simulink model "exercise1_Dengliang"  (R2024b)
settings: Solver=VariableStepAuto  StartTime=0.0  StopTime=20000  RelTol=1e-3
libraries: simulink x4
settings Model: Creator=10027  LastModifiedBy=10027

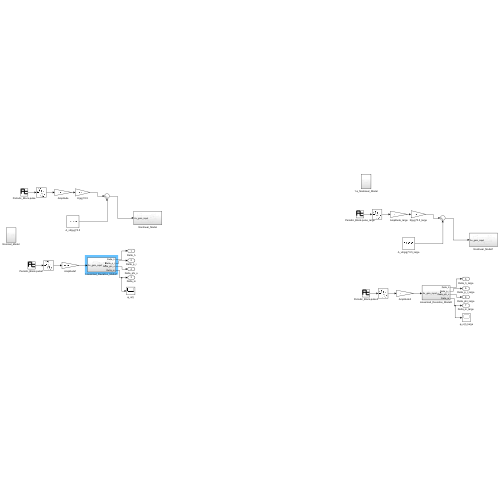
[thumbnail: Simulink's stored preview of the top-level diagram]
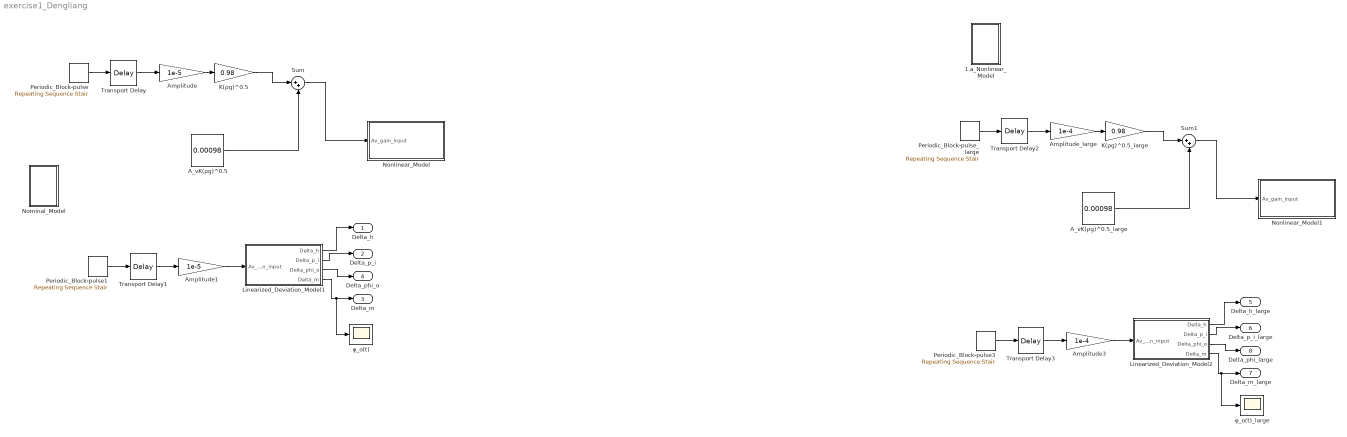
== system exercise1_Dengliang ==
  1.a_Nonlinear_Model : Subsystem
  A_vK(ρg)^0.5 : Constant  Value=0.00098
  A_vK(ρg)^0.5_large : Constant  Value=0.00098
  Amplitude : Gain  Gain=1e-5
  Amplitude1 : Gain  Gain=1e-5
  Amplitude3 : Gain  Gain=1e-4
  Amplitude_large : Gain  Gain=1e-4
  K(ρg)^0.5 : Gain  Gain=0.98
  K(ρg)^0.5_large : Gain  Gain=0.98
  Linearized_Deviation_Model1 : Subsystem
  Linearized_Deviation_Model2 : Subsystem
  Nominal_Model : Subsystem
  Nonlinear_Model : Subsystem
  Nonlinear_Model1 : Subsystem
  Periodic_Block-pulse : simulink/Sources/Repeating Sequence Stair  OutValues=[1 -1]  tsamp=3000  OutMin=[]  OutMax=[]  OutDataTypeStr=double  OutputDataTypeScalingMode=double  OutDataType=fixdt(0,8)  ConRadixGroup=Best Precision: Vector-wise  OutScaling=2^-12
  Periodic_Block-pulse1 : simulink/Sources/Repeating Sequence Stair  OutValues=[1 -1]  tsamp=3000  OutMin=[]  OutMax=[]  OutDataTypeStr=double  OutputDataTypeScalingMode=double  OutDataType=fixdt(0,8)  ConRadixGroup=Best Precision: Vector-wise  OutScaling=2^-12
  Periodic_Block-pulse3 : simulink/Sources/Repeating Sequence Stair  OutValues=[1 -1]  tsamp=3000  OutMin=[]  OutMax=[]  OutDataTypeStr=double  OutputDataTypeScalingMode=double  OutDataType=fixdt(0,8)  ConRadixGroup=Best Precision: Vector-wise  OutScaling=2^-12
  Periodic_Block-pulse_large : simulink/Sources/Repeating Sequence Stair  OutValues=[1 -1]  tsamp=3000  OutMin=[]  OutMax=[]  OutDataTypeStr=double  OutputDataTypeScalingMode=double  OutDataType=fixdt(0,8)  ConRadixGroup=Best Precision: Vector-wise  OutScaling=2^-12
  Sum : Sum  Inputs=|++
  Sum1 : Sum  Inputs=|++
  Transport Delay{,1..3} (4 alike) : TransportDelay  DelayTime=1000
  φ_o(t) : Scope
  φ_o(t)_large : Scope
  Delta_h : Outport
  Delta_p_i : Outport  Port=2
  Delta_m : Outport  Port=3
  Delta_phi_o : Outport  Port=4
  Delta_h_large : Outport  Port=5
  Delta_p_i_large : Outport  Port=6
  Delta_m_large : Outport  Port=7
  Delta_phi_large : Outport  Port=8
  wires:
  Periodic_Block-pulse/1 -> Transport Delay/1
  Amplitude/1 -> K(ρg)^0.5/1
  Transport Delay/1 -> Amplitude/1
  K(ρg)^0.5/1 -> Sum/1
  Sum/1 -> Nonlinear_Model/1(Av_gain_input)
  A_vK(ρg)^0.5/1 -> Sum/2
  Amplitude1/1 -> Linearized_Deviation_Model1/1(Av_gain_input)
  Periodic_Block-pulse1/1 -> Transport Delay1/1
  Transport Delay1/1 -> Amplitude1/1
  Linearized_Deviation_Model1/1(Delta_h) -> Delta_h/1
  Linearized_Deviation_Model1/2(Delta_p_i) -> Delta_p_i/1
  Linearized_Deviation_Model1/3(Delta_phi_o) -> Delta_phi_o/1
  Linearized_Deviation_Model1/4(Delta_m) -> φ_o(t)/1, Delta_m/1
  Amplitude3/1 -> Linearized_Deviation_Model2/1(Av_gain_input)
  Linearized_Deviation_Model2/1(Delta_h) -> Delta_h_large/1
  Periodic_Block-pulse3/1 -> Transport Delay3/1
  Transport Delay3/1 -> Amplitude3/1
  Linearized_Deviation_Model2/3(Delta_phi_o) -> Delta_phi_large/1
  K(ρg)^0.5_large/1 -> Sum1/1
  Sum1/1 -> Nonlinear_Model1/1(Av_gain_input)
  Periodic_Block-pulse_large/1 -> Transport Delay2/1
  Linearized_Deviation_Model2/4(Delta_m) -> φ_o(t)_large/1, Delta_m_large/1
  Linearized_Deviation_Model2/2(Delta_p_i) -> Delta_p_i_large/1
  Transport Delay2/1 -> Amplitude_large/1
  Amplitude_large/1 -> K(ρg)^0.5_large/1
  A_vK(ρg)^0.5_large/1 -> Sum1/2

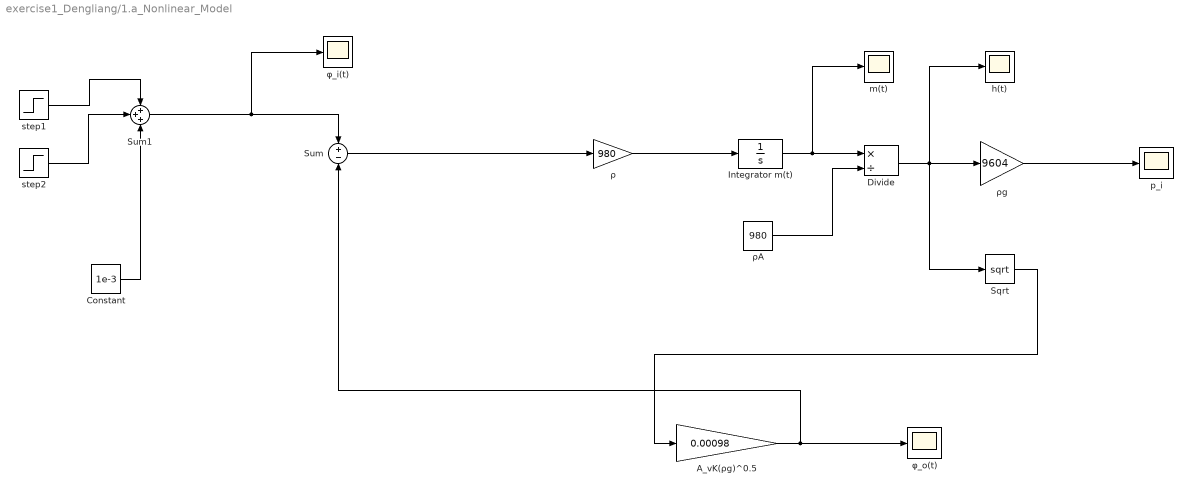
== system exercise1_Dengliang/1.a_Nonlinear_Model ==
  "A_vK(ρg)^0.5 " : Gain  Gain=0.00098
  Constant : Constant  Value=1e-3
  Divide : Product  Inputs=*/
  Integrator m(t) : Integrator  InitialCondition=1020.4
  Sqrt : Sqrt
  Sum : Sum  Inputs=+-
  Sum1 : Sum  Inputs=+++
  h(t) : Scope
  m(t) : Scope
  p_i : Scope
  step1 : Step  Time=2000  After=-0.5e-3  SampleTime=0
  step2 : Step  Time=12000  After=+0.5e-3  SampleTime=0
  ρ : Gain  Gain=980
  ρA : Constant  Value=980
  ρg : Gain  Gain=9604
  φ_i(t) : Scope
  φ_o(t) : Scope
  wires:
  ρg/1 -> p_i/1
  Integrator m(t)/1 -> m(t)/1, Divide/1
  Sum1/1 -> φ_i(t)/1, Sum/1
  Sum/1 -> ρ/1
  Sqrt/1 -> "A_vK(ρg)^0.5 "/1
  step1/1 -> Sum1/1
  Divide/1 -> h(t)/1, Sqrt/1, ρg/1
  ρA/1 -> Divide/2
  Constant/1 -> Sum1/3
  step2/1 -> Sum1/2
  ρ/1 -> Integrator m(t)/1
  "A_vK(ρg)^0.5 "/1 -> Sum/2, φ_o(t)/1

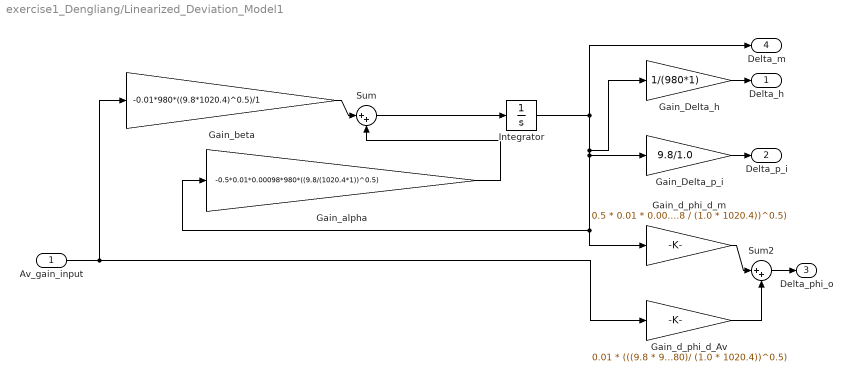
== system exercise1_Dengliang/Linearized_Deviation_Model1 ==
  Av_gain_input : Inport
  Gain_Delta_h : Gain  Gain=1/(980*1)
  Gain_Delta_p_i : Gain  Gain=9.8/1.0
  Gain_alpha : Gain  Gain=-0.5*0.01*0.00098*980*((9.8/(1020.4*1))^0.5)
  Gain_beta : Gain  Gain=-0.01*980*((9.8*1020.4)^0.5)/1
  Gain_d_phi_d_Av : Gain  Gain=0.01 * (((9.8 * 980)/ (1.0 * 1020.4))^0.5)
  Gain_d_phi_d_m : Gain  Gain=0.5 * 0.01 * 0.001 * ((9.8 / (1.0 * 1020.4))^0.5)
  Integrator : Integrator  ZeroCross=off
  Sum : Sum  Inputs=|++
  Sum2 : Sum  Inputs=|++
  Delta_h : Outport
  Delta_p_i : Outport  Port=2
  Delta_phi_o : Outport  Port=3
  Delta_m : Outport  Port=4
  wires:
  Av_gain_input/1 -> Gain_d_phi_d_Av/1, Gain_beta/1
  Integrator/1 -> Gain_alpha/1, Gain_d_phi_d_m/1, Gain_Delta_p_i/1, Gain_Delta_h/1, Delta_m/1
  Gain_Delta_h/1 -> Delta_h/1
  Gain_Delta_p_i/1 -> Delta_p_i/1
  Gain_d_phi_d_m/1 -> Sum2/1
  Gain_d_phi_d_Av/1 -> Sum2/2
  Sum2/1 -> Delta_phi_o/1
  Gain_beta/1 -> Sum/1
  Gain_alpha/1 -> Sum/2
  Sum/1 -> Integrator/1

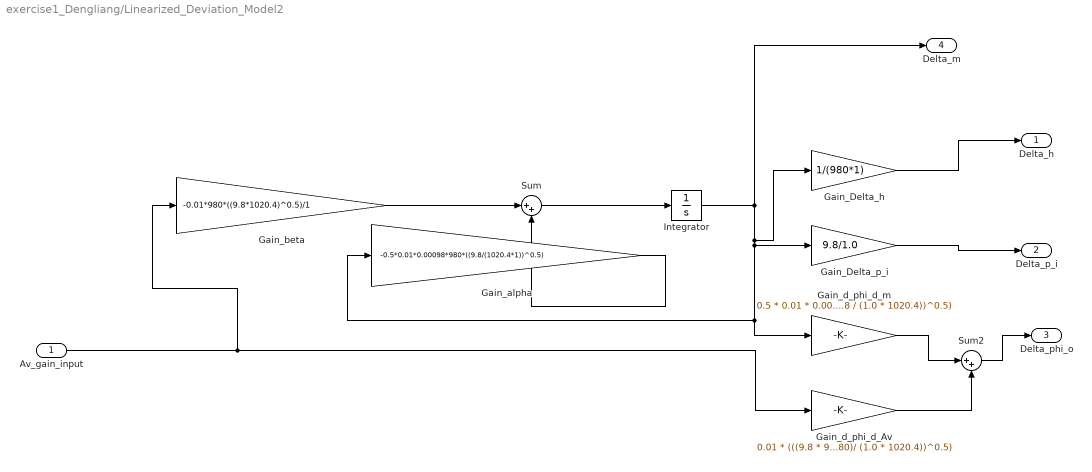
== system exercise1_Dengliang/Linearized_Deviation_Model2 ==
  Av_gain_input : Inport
  Gain_Delta_h : Gain  Gain=1/(980*1)
  Gain_Delta_p_i : Gain  Gain=9.8/1.0
  Gain_alpha : Gain  Gain=-0.5*0.01*0.00098*980*((9.8/(1020.4*1))^0.5)
  Gain_beta : Gain  Gain=-0.01*980*((9.8*1020.4)^0.5)/1
  Gain_d_phi_d_Av : Gain  Gain=0.01 * (((9.8 * 980)/ (1.0 * 1020.4))^0.5)
  Gain_d_phi_d_m : Gain  Gain=0.5 * 0.01 * 0.001 * ((9.8 / (1.0 * 1020.4))^0.5)
  Integrator : Integrator  ZeroCross=off
  Sum : Sum  Inputs=|++
  Sum2 : Sum  Inputs=|++
  Delta_h : Outport
  Delta_p_i : Outport  Port=2
  Delta_phi_o : Outport  Port=3
  Delta_m : Outport  Port=4
  wires:
  Av_gain_input/1 -> Gain_d_phi_d_Av/1, Gain_beta/1
  Integrator/1 -> Gain_alpha/1, Gain_d_phi_d_m/1, Gain_Delta_p_i/1, Gain_Delta_h/1, Delta_m/1
  Gain_Delta_h/1 -> Delta_h/1
  Gain_Delta_p_i/1 -> Delta_p_i/1
  Gain_d_phi_d_m/1 -> Sum2/1
  Gain_d_phi_d_Av/1 -> Sum2/2
  Sum2/1 -> Delta_phi_o/1
  Gain_beta/1 -> Sum/1
  Gain_alpha/1 -> Sum/2
  Sum/1 -> Integrator/1

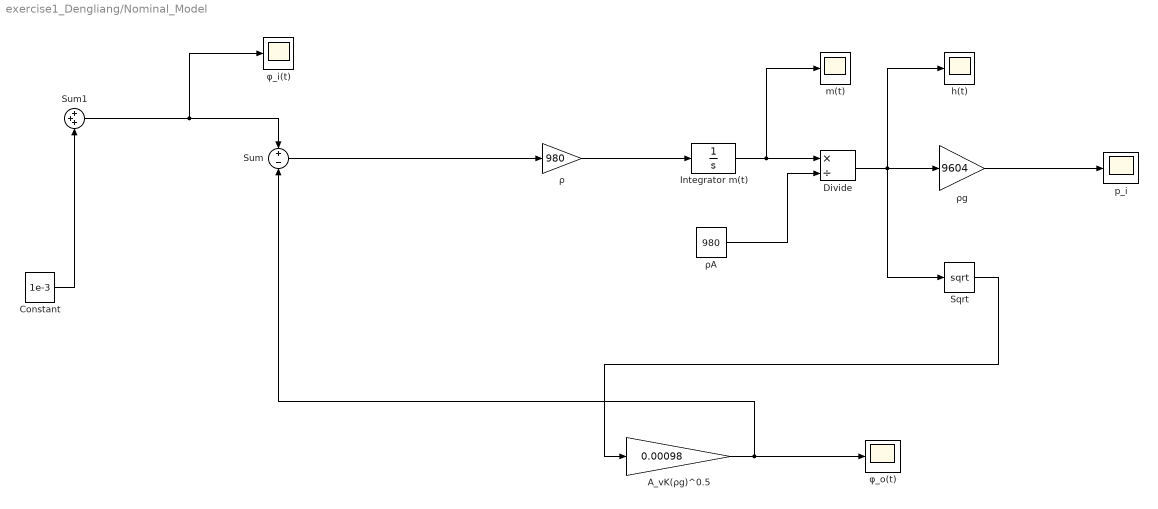
== system exercise1_Dengliang/Nominal_Model ==
  "A_vK(ρg)^0.5 " : Gain  Gain=0.00098
  Constant : Constant  Value=1e-3
  Divide : Product  Inputs=*/
  Integrator m(t) : Integrator  InitialCondition=1020.4
  Sqrt : Sqrt
  Sum : Sum  Inputs=+-
  Sum1 : Sum  Inputs=+++
  h(t) : Scope
  m(t) : Scope
  p_i : Scope
  ρ : Gain  Gain=980
  ρA : Constant  Value=980
  ρg : Gain  Gain=9604
  φ_i(t) : Scope
  φ_o(t) : Scope
  wires:
  ρg/1 -> p_i/1
  Integrator m(t)/1 -> m(t)/1, Divide/1
  Sum1/1 -> φ_i(t)/1, Sum/1
  Sum/1 -> ρ/1
  Sqrt/1 -> "A_vK(ρg)^0.5 "/1
  Divide/1 -> h(t)/1, Sqrt/1, ρg/1
  ρA/1 -> Divide/2
  Constant/1 -> Sum1/3
  ρ/1 -> Integrator m(t)/1
  "A_vK(ρg)^0.5 "/1 -> Sum/2, φ_o(t)/1

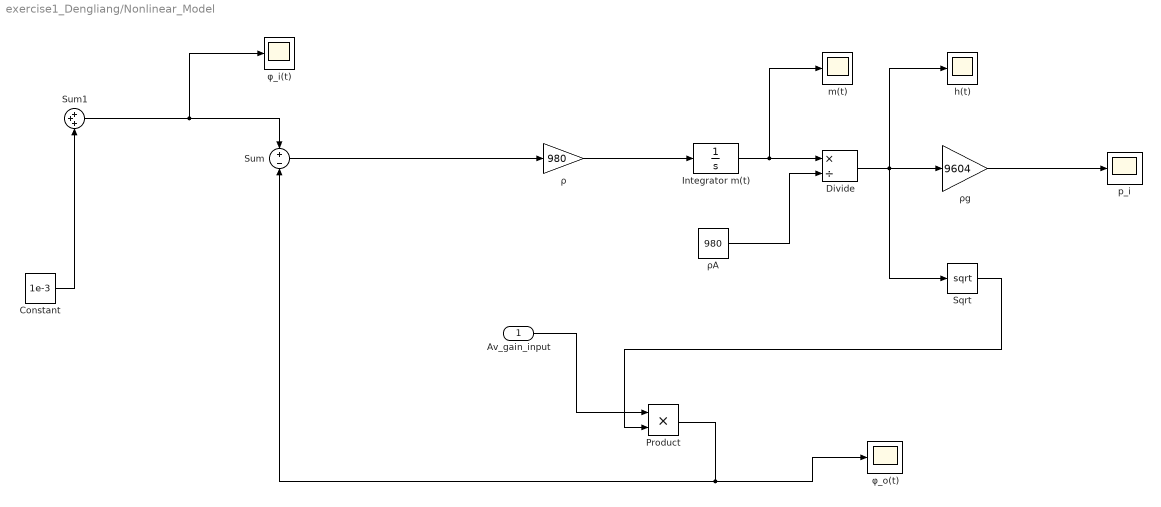
== system exercise1_Dengliang/Nonlinear_Model ==
  Av_gain_input : Inport
  Constant : Constant  Value=1e-3
  Divide : Product  Inputs=*/
  Integrator m(t) : Integrator  InitialCondition=1020.4
  Product : Product
  Sqrt : Sqrt
  Sum : Sum  Inputs=+-
  Sum1 : Sum  Inputs=+++
  h(t) : Scope
  m(t) : Scope
  p_i : Scope
  ρ : Gain  Gain=980
  ρA : Constant  Value=980
  ρg : Gain  Gain=9604
  φ_i(t) : Scope
  φ_o(t) : Scope
  wires:
  ρg/1 -> p_i/1
  Integrator m(t)/1 -> m(t)/1, Divide/1
  Sum1/1 -> φ_i(t)/1, Sum/1
  Sum/1 -> ρ/1
  Sqrt/1 -> Product/2
  Divide/1 -> h(t)/1, Sqrt/1, ρg/1
  ρA/1 -> Divide/2
  Constant/1 -> Sum1/3
  ρ/1 -> Integrator m(t)/1
  Av_gain_input/1 -> Product/1
  Product/1 -> φ_o(t)/1, Sum/2

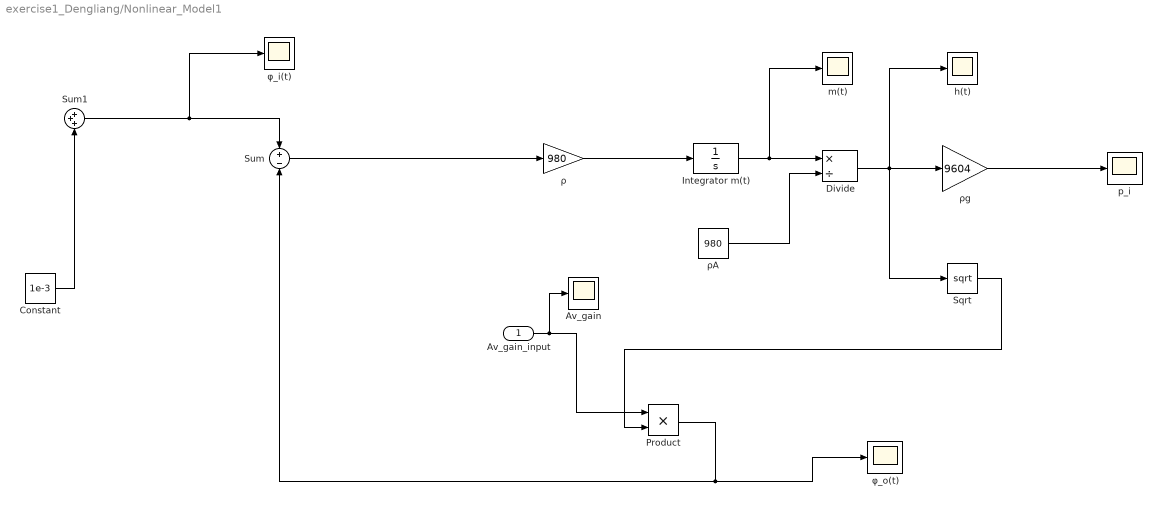
== system exercise1_Dengliang/Nonlinear_Model1 ==
  Av_gain_input : Inport
  Av_gain : Scope
  Constant : Constant  Value=1e-3
  Divide : Product  Inputs=*/
  Integrator m(t) : Integrator  InitialCondition=1020.4
  Product : Product
  Sqrt : Sqrt
  Sum : Sum  Inputs=+-
  Sum1 : Sum  Inputs=+++
  h(t) : Scope
  m(t) : Scope
  p_i : Scope
  ρ : Gain  Gain=980
  ρA : Constant  Value=980
  ρg : Gain  Gain=9604
  φ_i(t) : Scope
  φ_o(t) : Scope
  wires:
  ρg/1 -> p_i/1
  Integrator m(t)/1 -> m(t)/1, Divide/1
  Sum1/1 -> φ_i(t)/1, Sum/1
  Sum/1 -> ρ/1
  Sqrt/1 -> Product/2
  Divide/1 -> h(t)/1, Sqrt/1, ρg/1
  ρA/1 -> Divide/2
  Constant/1 -> Sum1/3
  ρ/1 -> Integrator m(t)/1
  Av_gain_input/1 -> Av_gain/1, Product/1
  Product/1 -> φ_o(t)/1, Sum/2
